simulink model "inner"  (R2023b)
settings: Solver=VariableStepAuto  StartTime=0.0  StopTime=10.0  RelTol=1e-3
model workspace (MATLAB code in the model file):
  | rho = 1.225;
  | R = 0.355;
  | omega_w = 3000;
  | K = rho*pi*R^2 * (omega_w*R)^2;
  | l = 0.4;
  | 
  | m = 12;
  | g = 9.81;
  | I = diag([1.86, 2.031, 3.617]);
  | 
  | zeta_x = diag([0.95, 0.95, 0.95]);
  | omega_n_x = diag([5, 5, 5]);
  | 
  | zeta_q = diag([0.95, 0.95, 0.95, 0.95]);
  | omega_n_q = diag([25, 25, 25, 25]);
  | 
  | V_tip           = omega_w * R;                        % Blade tip velocity in m/s
  | blade_area      = pi * R^2;                     % Blade area
  | CT_init         = (0.25*m*g/(rho*blade_area*V_tip^2));
settings Model: Creator=dsai9  LastModifiedBy=dsai9

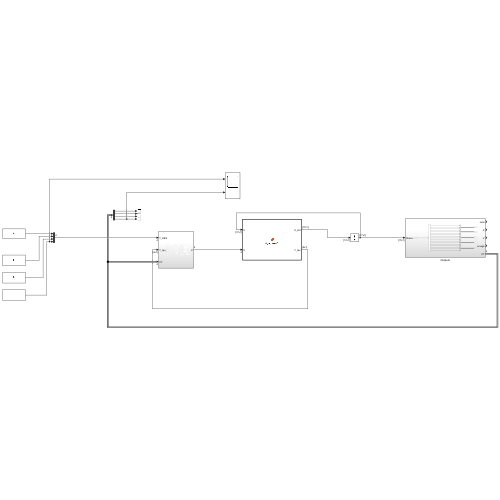
[thumbnail: Simulink's stored preview of the top-level diagram]
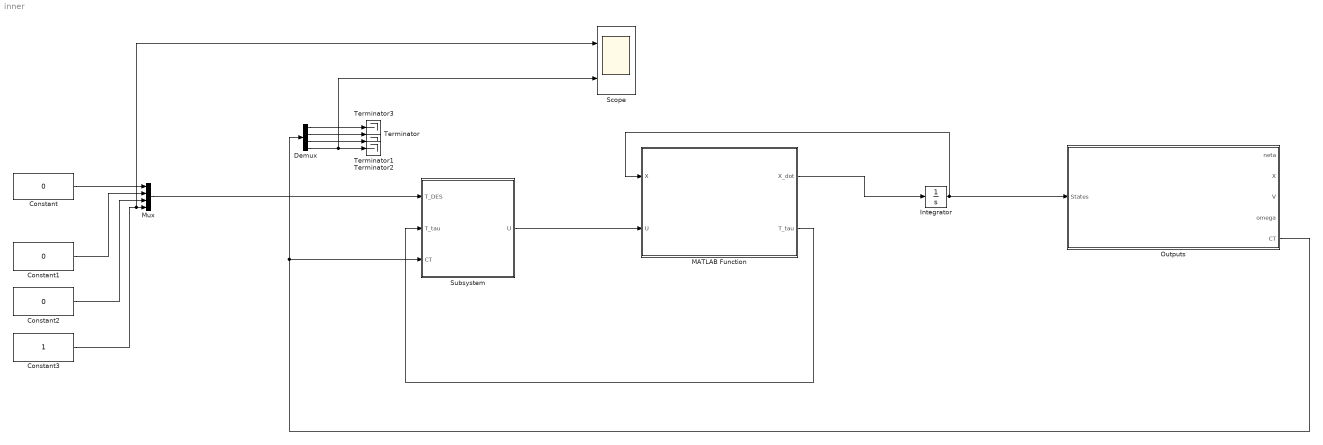
== system inner ==
  Constant : Constant  Value=0
  Constant1 : Constant  Value=0
  Constant2 : Constant  Value=0
  Constant3 : Constant
  Demux : Demux
  Integrator : Integrator  InitialCondition=[0; 0; 0; 0; 0; 0; 1; 0; 0; 0; 0; 0; 0; CT_init; CT_init; CT_init; CT_init]
  MATLAB Function : MATLAB Function  TreatAsAtomicUnit=on
  Mux : Mux
  Outputs : Subsystem
  Scope : Scope  NumInputPorts=2
  Subsystem : Subsystem
  Terminator{,1..3} (4 alike) : Terminator
  wires:
  MATLAB Function/1(X_dot) -> Integrator/1
  Integrator/1 -> MATLAB Function/1(X), Outputs/1(States)
  Outputs/5(CT) -> Demux/1, Subsystem/3(CT)
  Constant/1 -> Mux/1
  Constant1/1 -> Mux/2
  Mux/1 -> Subsystem/1(T_DES)
  Demux/2 -> Terminator/1
  Demux/3 -> Terminator1/1
  Demux/4 -> Scope/2, Terminator2/1
  Demux/1 -> Terminator3/1
  Constant2/1 -> Mux/3
  Constant3/1 -> Scope/1, Mux/4
  Subsystem/1(U) -> MATLAB Function/2(U)
  MATLAB Function/2(T_tau) -> Subsystem/2(T_tau)

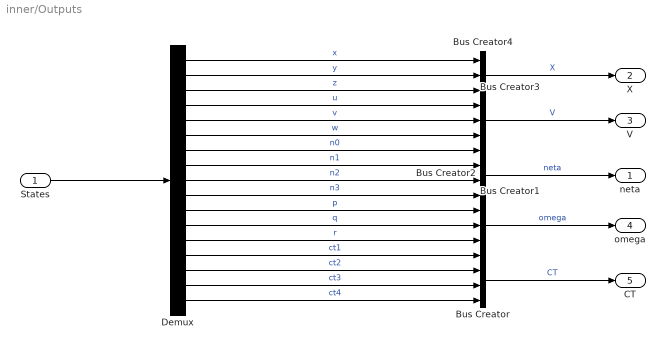
== system inner/Outputs ==
  States : Inport
  Bus Creator : BusCreator  Inputs=4
  Bus Creator1 : BusCreator  Inputs=3
  Bus Creator2 : BusCreator  Inputs=4
  Bus Creator3 : BusCreator  Inputs=3
  Bus Creator4 : BusCreator  Inputs=3
  Demux : Demux  Outputs=17
  neta : Outport
  X : Outport  Port=2
  V : Outport  Port=3
  omega : Outport  Port=4
  CT : Outport  Port=5
  wires:
  Demux/6 -> Bus Creator3/3  "w"
  Demux/3 -> Bus Creator4/3  "z"
  Demux/7 -> Bus Creator2/1  "n0"
  Bus Creator4/1 -> X/1  "X"
  Demux/16 -> Bus Creator/3  "ct3"
  Demux/17 -> Bus Creator/4  "ct4"
  Demux/10 -> Bus Creator2/4  "n3"
  Demux/14 -> Bus Creator/1  "ct1"
  Demux/15 -> Bus Creator/2  "ct2"
  Demux/13 -> Bus Creator1/3  "r"
  Demux/11 -> Bus Creator1/1  "p"
  Demux/2 -> Bus Creator4/2  "y"
  Demux/12 -> Bus Creator1/2  "q"
  Demux/9 -> Bus Creator2/3  "n2"
  Demux/8 -> Bus Creator2/2  "n1"
  Demux/5 -> Bus Creator3/2  "v"
  Demux/4 -> Bus Creator3/1  "u"
  Demux/1 -> Bus Creator4/1  "x"
  Bus Creator1/1 -> omega/1  "omega"
  Bus Creator/1 -> CT/1  "CT"
  Bus Creator3/1 -> V/1  "V"
  States/1 -> Demux/1
  Bus Creator2/1 -> neta/1  "neta"

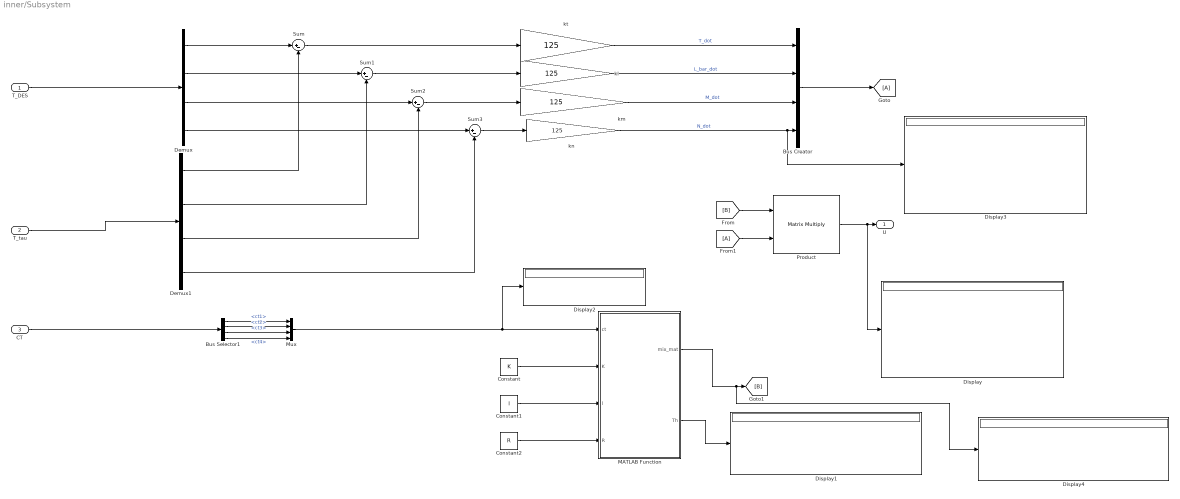
== system inner/Subsystem ==
  T_DES : Inport
  T_tau : Inport  Port=2
  CT : Inport  Port=3
  Bus Creator : BusCreator  Inputs=4
  Bus Selector1 : BusSelector  OutputSignals=ct1,ct2,ct3,ct4
  Constant : Constant  Value=K
  Constant1 : Constant  Value=l
  Constant2 : Constant  Value=R
  Demux : Demux
  Demux1 : Demux
  Display{,1..4} (5 alike) : Display
  From1 : From
  Goto : Goto
  MATLAB Function : MATLAB Function  TreatAsAtomicUnit=on
  Mux : Mux
  Product : Product  Multiplication=Matrix(*)
  Sum{,1..3} (4 alike) : Sum  Inputs=|+-
  kl : Gain  Gain=125
  km : Gain  Gain=125
  kn : Gain  Gain=125
  kt : Gain  Gain=125
  U : Outport
  wires:
  T_tau/1 -> Demux1/1
  T_DES/1 -> Demux/1
  Demux/1 -> Sum/1
  Demux1/1 -> Sum/2
  Demux/2 -> Sum1/1
  Demux1/2 -> Sum1/2
  Demux/3 -> Sum2/1
  Demux1/3 -> Sum2/2
  Demux/4 -> Sum3/1
  Demux1/4 -> Sum3/2
  Sum/1 -> kt/1
  Sum1/1 -> kl/1
  Sum2/1 -> km/1
  Sum3/1 -> kn/1
  kl/1 -> Bus Creator/2  "L_bar_dot"
  km/1 -> Bus Creator/3  "M_dot"
  kn/1 -> Display3/1, Bus Creator/4  "N_dot"
  kt/1 -> Bus Creator/1  "T_dot"
  Constant/1 -> MATLAB Function/2(K)
  Constant1/1 -> MATLAB Function/3(l)
  Constant2/1 -> MATLAB Function/4(R)
  CT/1 -> Bus Selector1/1
  Bus Selector1/1 -> Mux/1  "<ct1>"
  Bus Selector1/2 -> Mux/2  "<ct2>"
  Bus Selector1/3 -> Mux/3  "<ct3>"
  Bus Selector1/4 -> Mux/4  "<ct4>"
  Mux/1 -> Display2/1, MATLAB Function/1(ct)
  Bus Creator/1 -> Goto/1
  MATLAB Function/1(mix_mat) -> Display4/1, [B]
  [B] -> Product/1
  From1/1 -> Product/2
  Product/1 -> Display/1, U/1
  MATLAB Function/2(Th) -> Display1/1

== matlab function inner/Subsystem/MATLAB Function ==
  data: ct input; mix_mat output; K input; l input; R input; Th output
function [mix_mat, Th] = fcn(ct, K, l, R)
ct1 = ct(1);
ct2 = ct(2);
ct3 = ct(3);
ct4 = ct(4);

Th = [K K K K ; K*l -K*l -K*l K*l; K*l K*l -K*l -K*l; 
    (3*K*R/2)*sqrt(abs(ct1)/2) -(3*K*R/2)*sqrt(abs(ct2)/2) (3*K*R/2)*sqrt(abs(ct3)/2) -(3*K*R/2)*sqrt(abs(ct4)/2)];

mix_mat = pinv(Th);

== matlab function inner/MATLAB Function ==
  settings: updateMethod=DISCRETE  sampleTime=0.01
  data: X input double size=[17,1]; X_dot output double size=[17,1]; U input double size=[4,1]; T_tau output
function [X_dot, T_tau] = dynamics2(X,U)

% k_t = 1e-3; % Thrust Coefficient

%% Parameters
m               = 12;                       % Mass in kg
g               = 9.81;   
l               = 0.40;                         % Arm length in m
rho = 1.225;
R               = 0.355;   
omega_w = 3000;
K               = rho * pi * R^2 * (omega_w * R)^2;



I = diag([1.86, 2.031, 3.617]);
I_x = I(1,1);
I_y = I(2,2);
I_z = I(3,3);
I_xz = 0;


%% State Unpacking
% w1 = u(1);
% w2 = u(2);
% w3 = u(3);
% w4 = u(4);



% Linear Velocity
u = X(4);
v = X(5);
w = X(6);

% Orientation In Quaternion
n0 = X(7);
n1 = X(8);
n2 = X(9);
n3 = X(10);

% Angular Velocity
p = X(11);
q = X(12);
r = X(13);

% Thrust Coefficients
ct1 = X(14);
ct2 = X(15);
ct3 = X(16);
ct4 = X(17);

%% Aero Dynamic Forces (TBD)
F_ax = 0;
F_ay = 0;
F_az = 0;

L_abar = 0;
% L_tbar = 0;
M_a = 0;
% M_t = 0;
N_a = 0;
% N_t = 0;


%% Constants
C1 = (1/(I_x*I_z - I_xz)) .* [(I_y - I_z)*I_z - I_xz^2;
                             (I_x - I_y + I_z)*I_xz;
                             I_z;
                             I_xz;
                             (I_x - I_y)*I_x + I_xz^2;
                             I_x];
c1 = C1(1);
c2 = C1(2);
c3 = C1(3);
c4 = C1(4);
c8 = C1(5);
c9 = C1(6);

C2 = (1/I_y) .*  [(I_z - I_x);
                  I_xz;
                  1];

c5 = C2(1);
c6 = C2(2);
c7 = C2(3);

%% Control Allocation
T = K*(ct1 + ct2 + ct3 + ct4);
L_tbar = K * l *(ct1 - ct2 - ct3 + ct4);
M_t = K * l * (ct1 + ct2 - ct3 - ct4);
N_t = (K*R/sqrt(2)) * (abs(ct1)^1.5 - abs(ct2)^1.5 + abs(ct3)^1.5 - abs(ct4)^1.5);
%% True Air Speed and Dynamic Pressure
% rho = 1.225;
% V = sqrt(u^2 + v^2 + w^2);
% Q_inf = 0.5*rho*V^2;


% Rotation Matrices
Rot_mat_body2iner_inquat = [n0^2+n1^2-n2^2-n3^2, (2*n1*n2)-(2*n3*n0), (2*n1*n3) + (2*n2*n0);
                     (2*n1*n2)+(2*n3*n0), (n0^2-n1^2+n2^2-n3^2), (2*n2*n3)-(2*n0*n1);
                     (2*n1*n3)-(2*n2*n0), (2*n2*n3+2*n1*n0), (n0^2-n1^2-n2^2+n3^2)];

%% Dynamics
% T = k_t*(w1^2 + w2^2 + w3^2 + w4^2);
lin_vel_dot = [0; 0; -T/m] + [F_ax/m; F_ay/m; F_az/m] +g .* [2*n1*n3 - 2*n0*n2; 2*n2*n3 + 2*n0*n1; n0^2-n1^2-n2^2+n3^2] + [r*v - q*w; p*w - r*u; q*u - p*v];
ang_vel_dot = [(c1*r + c2*p)*q + c3*(L_abar + L_tbar) + c4*(N_a + N_t);
                c5*p*r - c6*(p^2 - r^2) + c7*(M_a + M_t);
                (c8*p - c2*r)*q + c4*(L_abar + L_tbar) + c9*(N_a + N_t)];

%% Kinematics 
pos_dot = Rot_mat_body2iner_inquat*[u; v; w];
n_dot = 0.5 .* [-n1, -n2, -n3;
                n0, -n3, n2;
                n3, n0, -n1;
                -n2, n1, n0] * [p; q; r];

%% Inputs
ct_dot = U;

T_tau = [T; L_tbar; M_t; N_t];

X_dot = [pos_dot; lin_vel_dot; n_dot; ang_vel_dot; ct_dot];
